simulink model "mlf_sample1"  (R2015b)
settings: Solver=FixedStepDiscrete  SolverMode=SingleTasking  StartTime=0.0  StopTime=4  RelTol=1e-3
libraries: simulink x1
settings Model: Creator=at-mt  LastModifiedBy=amatsumo
settings DataIOCC: SaveFormat=Array  SignalLoggingSaveFormat=ModelDataLogs  SaveOutput=off  SignalLogging=off  SaveTime=off
settings OptimizationCC: BlockReduction=off  ConditionallyExecuteInputs=off  DefaultParameterBehavior=Inlined  ExpressionDepthLimit=2147483647
settings DebuggingCC: AlgebraicLoopMsg=error  UnderspecifiedInitializationDetection=Classic  MergeDetectMultiDrivingBlocksExec=none  SolverPrmCheckMsg=warning  SingleTaskRateTransMsg=error  FcnCallInpInsideContextMsg=UseLocalSettings  StateNameClashWarn=warning
settings HardwareCC: ProdBitPerPointer=32  ProdLargestAtomicFloat=None  ProdIntDivRoundTo=Undefined  ProdEndianess=Unspecified  ProdWordSize=32  ProdHWDeviceType=ASIC/FPGA->ASIC/FPGA  ProdEqTarget=off
settings GRTTargetCC: GeneratePreprocessorConditionals=Disable all  CombineOutputUpdateFcns=off  GRTInterface=on
settings ConfigComp: CovModelRefEnable=Off  CovSFcnEnable=off

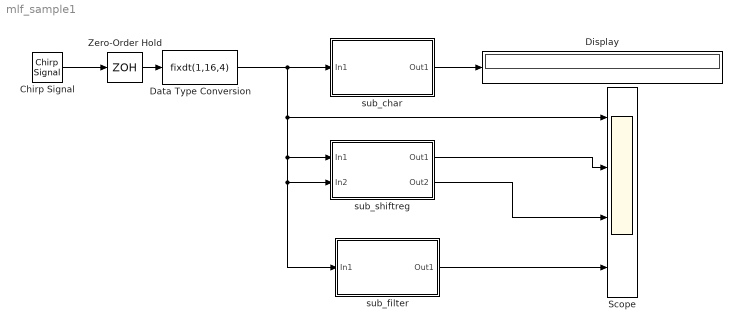
== system mlf_sample1 ==
  Chirp Signal : simulink/Sources/Chirp Signal  f1=10  T=10  f2=500
  Data Type Conversion : DataTypeConversion  OutDataTypeStr=fixdt(1,16,4)
  Display : Display
  Scope : Scope  NumInputPorts=4
  Zero-Order Hold : ZeroOrderHold  SampleTime=1/1000
  sub_char : Subsystem
  sub_filter : Subsystem
  sub_shiftreg : Subsystem
  wires:
  Chirp Signal/1 -> Zero-Order Hold/1
  Zero-Order Hold/1 -> Data Type Conversion/1
  Data Type Conversion/1 -> sub_char/1(In1), Scope/1, sub_shiftreg/1(In1), sub_filter/1(In1), sub_shiftreg/2(In2)
  sub_char/1(Out1) -> Display/1
  sub_shiftreg/1(Out1) -> Scope/2
  sub_filter/1(Out1) -> Scope/4
  sub_shiftreg/2(Out2) -> Scope/3

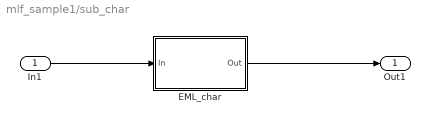
== system mlf_sample1/sub_char ==
  In1 : Inport
  EML_char : MATLAB Function  TreatAsAtomicUnit=on
  Out1 : Outport
  wires:
  In1/1 -> EML_char/1(In)
  EML_char/1(Out) -> Out1/1

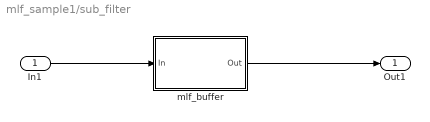
== system mlf_sample1/sub_filter ==
  In1 : Inport
  mlf_buffer : MATLAB Function  TreatAsAtomicUnit=on
  Out1 : Outport
  wires:
  mlf_buffer/1(Out) -> Out1/1
  In1/1 -> mlf_buffer/1(In)

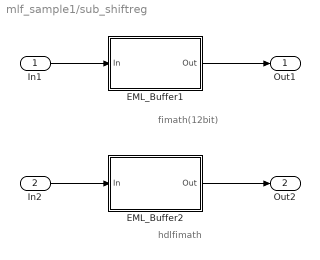
== system mlf_sample1/sub_shiftreg ==
  note: hdlfimath
  note: fimath(12bit)
  In1 : Inport
  In2 : Inport  Port=2
  EML_Buffer1 : MATLAB Function  TreatAsAtomicUnit=on
  EML_Buffer2 : MATLAB Function  TreatAsAtomicUnit=on
  Out1 : Outport
  Out2 : Outport  Port=2
  wires:
  EML_Buffer1/1(Out) -> Out1/1
  In1/1 -> EML_Buffer1/1(In)
  In2/1 -> EML_Buffer2/1(In)
  EML_Buffer2/1(Out) -> Out2/1

== matlab function mlf_sample1/sub_shiftreg/EML_Buffer2 ==
  settings: fimath=hdlfimath;
  data: In input; Out output
function Out = fcn(In)
% shift register 


persistent buf
if isempty(buf)
	% initialize register with zero data
	buf = fi(zeros(1,10),1,16,14);
end

% data shift
buf(2:end)=buf(1:end-1);

% input data
buf(1)=In;

Out = fi(1.2,1,16,14)*buf(end);

== matlab function mlf_sample1/sub_char/EML_char ==
  settings: fimath=|
      | fimath(...
      | 'RoundMode', 'floor',...
      | 'OverflowMode', 'wrap',...
      | 'ProductMode', 'KeepLSB', 'ProductWordLength', 16,...
      | 'SumMode', 'KeepLSB', 'SumWordLength', 16,...
      | 'CastBeforeSum', true)
  data: In input; Out output
function Out = fcn(In)
% This block supports the Embedded MATLAB subset.
% See the help menu for details. 
% Parameters

Data = char('aaa');


Out = int8(Data);

== matlab function mlf_sample1/sub_filter/mlf_buffer ==
  settings: fimath=|
      | fimath(...
      | 'RoundMode', 'floor',...
      | 'OverflowMode', 'wrap',...
      | 'ProductMode', 'KeepLSB', 'ProductWordLength', 16,...
      | 'SumMode', 'KeepLSB', 'SumWordLength', 16,...
      | 'CastBeforeSum', true)
  data: In input; Out output
function Out = fcn(In)
% shift register 

persistent buf
if isempty(buf)
	% initialize register with zero data
	buf = fi(zeros(1,5),1,16,14);
end

% data shift
buf(2:end)=buf(1:end-1);

% input data
buf(1)=In;

Out = sum(buf)*0.2;

== matlab function mlf_sample1/sub_shiftreg/EML_Buffer1 ==
  settings: fimath=|
      | fimath(...
      | 'RoundMode', 'floor',...
      | 'OverflowMode', 'wrap',...
      | 'ProductMode', 'KeepMSB', 'ProductWordLength', 12,...
      | 'SumMode', 'KeepMSB', 'SumWordLength', 12,...
      | 'CastBeforeSum', true)
  data: In input; Out output
function Out = fcn(In)
% shift register 


persistent buf
if isempty(buf)
	% initialize register with zero data
	buf = fi(zeros(1,10),1,16,14);
end

% data shift
buf(2:end)=buf(1:end-1);

% input data
buf(1)=In;

Out = fi(1.2,1,16,14)*buf(end);
